simulink model "all_in_one"  (R2024a)
settings: Solver=VariableStepAuto  StartTime=0.0  StopTime=2.5  RelTol=1e-3
settings Model: Creator=ericliu  LastModifiedBy=Eason

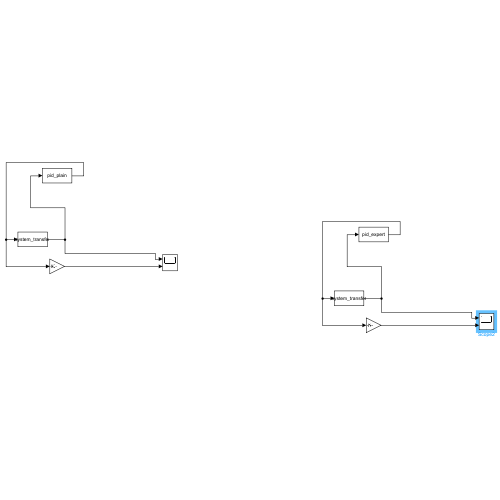
[thumbnail: Simulink's stored preview of the top-level diagram]
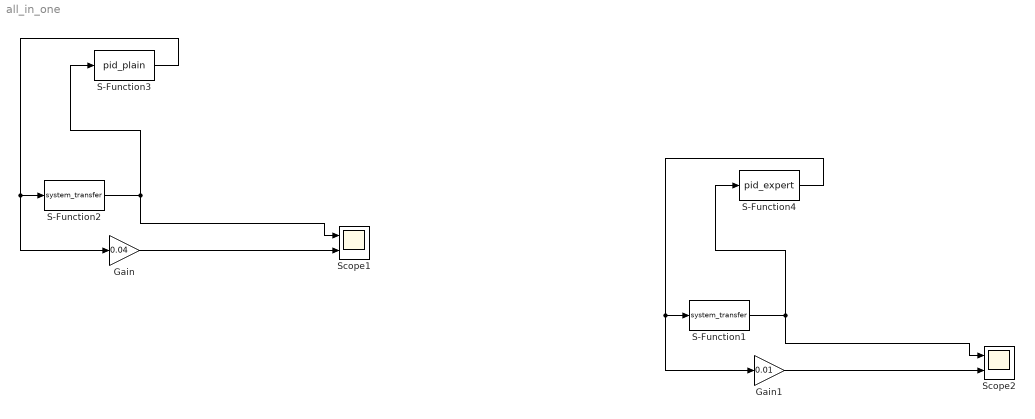
== system all_in_one ==
  Gain : Gain  Gain=0.04
  Gain1 : Gain  Gain=0.01
  S-Function1 : S-Function  FunctionName=system_transfer  SFunctionDeploymentMode=off  EnableBusSupport=off
  S-Function2 : S-Function  FunctionName=system_transfer  SFunctionDeploymentMode=off  EnableBusSupport=off
  S-Function3 : S-Function  FunctionName=pid_plain  SFunctionDeploymentMode=off  EnableBusSupport=off
  S-Function4 : S-Function  FunctionName=pid_expert  SFunctionDeploymentMode=off  EnableBusSupport=off
  Scope1 : Scope  NumInputPorts=2
  Scope2 : Scope  NumInputPorts=2
  wires:
  S-Function3/1 -> Gain/1, S-Function2/1
  S-Function2/1 -> S-Function3/1, Scope1/1
  Gain/1 -> Scope1/2
  S-Function4/1 -> Gain1/1, S-Function1/1
  S-Function1/1 -> S-Function4/1, Scope2/1
  Gain1/1 -> Scope2/2
